simulink model "Problem_4"  (R2020b)
settings: Solver=VariableStepAuto  StartTime=0.0  StopTime=10.0  RelTol=1e-3
settings Model: Creator=Yeshwanth  LastModifiedBy=Yeshwanth

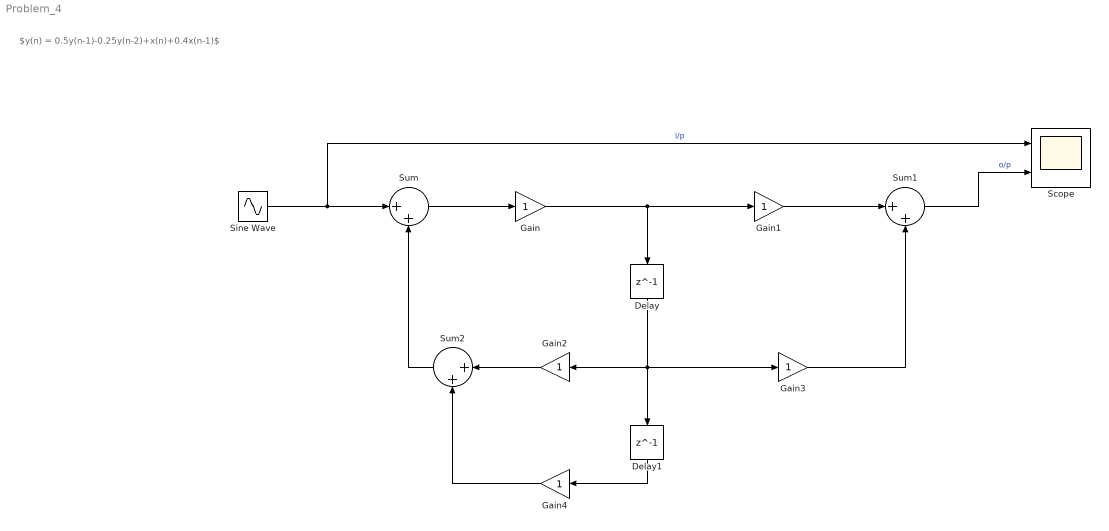
== system Problem_4 ==
  note: $y(n) = 0.5y(n-1)-0.25y(n-2)+x(n)+0.4x(n-1)$
  Delay : Delay  DelayLength=1
  Delay1 : Delay  DelayLength=1
  Gain{,1..4} (5 alike) : Gain
  Scope : Scope  NumInputPorts=2
  Sine Wave : Sin  SampleTime=0
  Sum : Sum  Inputs=|++
  Sum1 : Sum  Inputs=|++
  Sum2 : Sum  Inputs=|++
  wires:
  Sine Wave/1 -> Scope/1, Sum/1  "i/p"
  Sum1/1 -> Scope/2  "o/p"
  Sum/1 -> Gain/1
  Gain/1 -> Delay/1, Gain1/1
  Gain3/1 -> Sum1/2
  Gain1/1 -> Sum1/1
  Gain4/1 -> Sum2/2
  Gain2/1 -> Sum2/1
  Delay/1 -> Gain3/1, Gain2/1, Delay1/1
  Delay1/1 -> Gain4/1
  Sum2/1 -> Sum/2
